simulink model "LocalizationTest"  (R2023b)
settings: Solver=VariableStepAuto  StartTime=0.0  StopTime=2  RelTol=1e-3
settings Model: Creator=megan  LastModifiedBy=megan

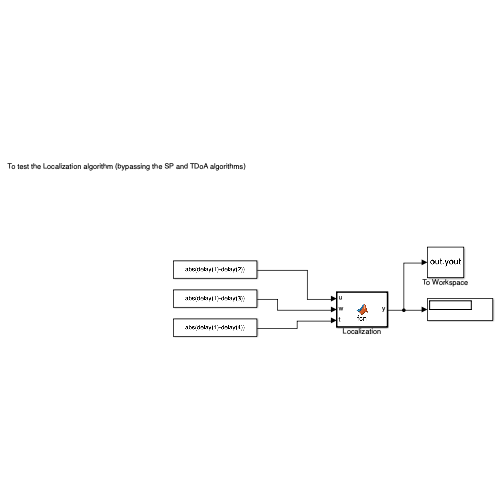
[thumbnail: Simulink's stored preview of the top-level diagram]
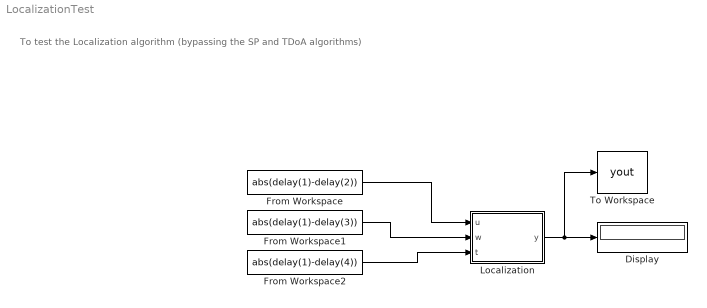
== system LocalizationTest ==
  note: To test the Localization algorithm (bypassing the SP and TDoA algorithms)
  Display : Display
  From Workspace : FromWorkspace  VariableName=abs(delay(1)-delay(2))
  From Workspace1 : FromWorkspace  VariableName=abs(delay(1)-delay(3))
  From Workspace2 : FromWorkspace  VariableName=abs(delay(1)-delay(4))
  Localization : MATLAB Function  TreatAsAtomicUnit=on
  To Workspace : ToWorkspace  VariableName=yout  SampleTime=-1
      settings: Save2DSignal=2-D array (concatenate along first dimension)
  wires:
  Localization/1(y) -> To Workspace/1, Display/1
  From Workspace/1 -> Localization/1(u)
  From Workspace1/1 -> Localization/2(w)
  From Workspace2/1 -> Localization/3(t)

== matlab function LocalizationTest/Localization ==
  data: u input; y output; w input; t input
function y = fcn(u, w, t)

y = u + w + t;
